simulink model "lateral_dyn_unconstrained"  (R2020b)
settings: Solver=VariableStepAuto  StartTime=0.0  StopTime=10.0  RelTol=1e-3
settings Model: Creator=User  LastModifiedBy=Matthew

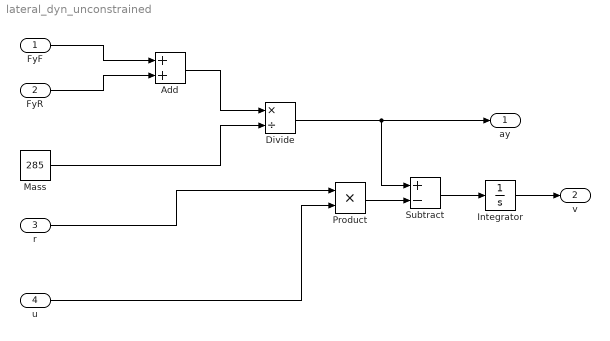
== system lateral_dyn_unconstrained ==
  FyF : Inport
  FyR : Inport  Port=2
  r : Inport  Port=3
  u : Inport  Port=4
  Add : Sum
  Divide : Product  Inputs=*/
  Integrator : Integrator
  Mass : Constant  Value=285
  Product : Product
  Subtract : Sum  Inputs=+-
  ay : Outport
  v : Outport  Port=2
  wires:
  FyF/1 -> Add/1
  Add/1 -> Divide/1
  Mass/1 -> Divide/2
  Divide/1 -> ay/1, Subtract/1
  Integrator/1 -> v/1
  FyR/1 -> Add/2
  u/1 -> Product/2
  Subtract/1 -> Integrator/1
  Product/1 -> Subtract/2
  r/1 -> Product/1
